simulink model "SIMULINK_ADP_Tracking_R2022b"  (R2023b)
settings: Solver=FixedStepAuto  StartTime=0.0  StopTime=sim_end_time  FixedStep=fixed_step_size  RelTol=1e-3
InitFcn:
  | start_uav_car_10
undefined symbols (not defined in the file): a, act_end, b, battery_threshold, bb, delta_, draw_gif, droneyeeUAV2_NUM, droneyeeUAV3_NUM, droneyeeUAV4_NUM, droneyeeUAV5_NUM, fixed_step_size, k, KD_x, KD_y, kd_z, KDD_x, KDD_y, KI_x, KI_y, ki_z, KII_x, KII_y, KP_x, KP_y, kp_z, KPP_x, KPP_y, lmt, omega, omega_, R, sim_end_time, uav10num, uav1num, uav2num, uav3num, uav4num, uav5num, uav6num, uav7num, uav8num, uav9num, UAV_NUM, Vel_Switch_1, Vel_Switch_10, Vel_Switch_11, Vel_Switch_12, Vel_Switch_13, Vel_Switch_14, Vel_Switch_15, Vel_Switch_16, Vel_Switch_17, Vel_Switch_18, Vel_Switch_19, Vel_Switch_2, Vel_Switch_20, Vel_Switch_3, Vel_Switch_4, Vel_Switch_5 ... (+15)
libraries: simulink x118, aerolibanimutils x1
(part 10 of 11)

== system SIMULINK_ADP_Tracking_R2022b/control system_UAV/Baseline Controller1/Position controller/X-Y ADP tracking controller ==
  Feedback1 : Inport
  Joystick : Inport  Port=2
  p_virtual : Inport  Port=3
  Clock1 : Clock
  Clock2 : Clock
  Clock3 : Clock
  Constant : Constant  Value=5
  Constant1 : Constant  Value=ys_learned
  DMP_ref : MATLAB Function  TreatAsAtomicUnit=on
  Delay : Delay  DelayLength=1  InitialCondition=delta_
  Delay1 : Delay  DelayLength=1  InitialCondition=omega_
  Demux : Demux  Outputs=2
  Demux1 : Demux  Outputs=2
  Derivative : Derivative
  Integrator : Integrator  InitialCondition=W0
  Integrator2 : Integrator  InitialCondition=zeros(2,1)
  Mux1 : Mux  Inputs=3
  Obstacle detection : MATLAB Function  TreatAsAtomicUnit=on
  Saturation : Saturate  UpperLimit=500  LowerLimit=-500
  Saturation1 : Saturate  UpperLimit=100  LowerLimit=-100
  Scope{,1,3..4,6} (5 alike) : Scope
  Scope2 : Scope  NumInputPorts=2
  Scope5 : Scope  NumInputPorts=2
  Terminator : Terminator
  Terminator1 : Terminator
  To Workspace1 : ToWorkspace  VariableName=W  SaveFormat=Timeseries  SampleTime=-1
  To Workspace2 : ToWorkspace  VariableName=Cache1  SampleTime=-1
  XY Graph : Record  FileSettingsInternal="{\"entries\":[{\"content\":{\"excelSettings\":{\"content\":{},\"type\":\"Streamout.ExcelSettings\"}},\"type\":\"Streamout.FileSettingStorage\",\"uuid\":\"\"}],\"packageUris\":[\"http:\\/\\/schema.mathworks.com\\/mf0\\/streamout_blocks\\/R2020a\"],\"version\":\"1.0\"}"  Layout=[1 1]  SignalsInternal="{\"entries\":[{\"content\":{\"signals\":[{\"content\":{\"blockPath\":[],\"dimensions\":[1,1],\"domain\":\"\",\"lineColor\":\"#edb120\",\"port\":1,\"signalID\":1,\"signalName\":\"Demux:1\"},\"type\":\"RecordBlkView.Signal\",\"uuid\":\"\"},{\"content\":{\"blockPath\":[],\"dimensions\":[1,1],\"domain\":\"\",\"lineColor\":\"#7e2f8e\",\"port\":2,\"signalID\":2,\"signalName\":\"Demux:2\"},\"type\":\"RecordBlkView.Signal\",\"uuid\":\"\"}]},\"type\":\"RecordBlkView.InputSignals\",\"uuid\":\"\"}],\"packageUris\":[\"http:\\/\\/schema.mathworks.com\\/mf0\\/streamout_blocks\\/R2020a\"],\"version\":\"1.0\"}"  VisualizationBindings="{\"xyplotplugin\":{\"info\":[{\"series\":[],\"subplotID\":1}]}}"  CompatibilityTag=XY
  adp_tracking : MATLAB Function  TreatAsAtomicUnit=on
  planning output : Scope  NumInputPorts=2
  reference_traj : MATLAB Function  TreatAsAtomicUnit=on
  ux : Outport
  uy : Outport  Port=2
  " p_virtual1" : Outport  Port=3
  wires:
  adp_tracking/1(ux1) -> Scope2/1, ux/1
  Obstacle detection/2(Cache1) -> To Workspace2/1
  Joystick/1 -> adp_tracking/3(Joystick)
  adp_tracking/3(delta_) -> Delay/1
  Delay/1 -> adp_tracking/4(delta_his)
  adp_tracking/4(omega_) -> Scope/1, Delay1/1
  Delay1/1 -> adp_tracking/5(omega_his)
  adp_tracking/5(dW_) -> Saturation/1
  Clock1/1 -> adp_tracking/7(t)
  Integrator/1 -> Scope1/1, To Workspace1/1, adp_tracking/6(W)
  Derivative/1 -> adp_tracking/8(dP_feedback1)
  Saturation/1 -> Integrator/1
  adp_tracking/6(test) -> Scope3/1
  Saturation1/1 -> Derivative/1
  Obstacle detection/1(y) -> Scope4/1, adp_tracking/9(lcoa)
  Demux/1 -> Mux1/1, XY Graph/1, Scope5/1
  Demux/2 -> Mux1/2, XY Graph/2, Scope5/2
  Mux1/1 -> " p_virtual1"/1
  Constant/1 -> Mux1/3
  adp_tracking/2(uy1) -> Scope2/2, uy/1
  reference_traj/1(dp_ref) -> Integrator2/1
  Integrator2/1 -> Terminator/1, reference_traj/2(p_ref)
  Clock2/1 -> reference_traj/1(t)
  reference_traj/2(u_adp) -> Demux1/1
  Demux1/1 -> planning output/1
  Demux1/2 -> planning output/2
  Constant1/1 -> DMP_ref/2(u)
  Clock3/1 -> DMP_ref/1(t)
  Feedback1/1 -> Obstacle detection/1(X), Saturation1/1, adp_tracking/1(P_feedback1)
  p_virtual/1 -> Demux/1, adp_tracking/2(p_virtual1), Scope6/1
  DMP_ref/1(y) -> Terminator1/1

== matlab function SIMULINK_ADP_Tracking_R2022b/control system_car1/Baseline Controller7/MATLAB Function ==
  data: u input; y output; a input
function y = fcn(u,a)
y = satgd(u,a);

== matlab function SIMULINK_ADP_Tracking_R2022b/control system_car1/Baseline Controller8/MATLAB Function ==
  data: u input; y output; a input
function y = fcn(u,a)
y = satgd(u,a);

== matlab function SIMULINK_ADP_Tracking_R2022b/control system_car1/Baseline Controller9/MATLAB Function ==
  data: u input; y output; a input
function y = fcn(u,a)
y = satgd(u,a);

== matlab function SIMULINK_ADP_Tracking_R2022b/防碰撞1/MATLAB Function1 ==
  settings: updateMethod=DISCRETE
  data: u1 input; xd output; u2 input; yd output; zd output; u3 input; u4 input; u5 input; flag input
function [xd,yd,zd] = fcn(u1,u2,u3,u4,u5,flag)

persistent xdd ydd zdd xtt ytt ztt;
k=u4;
totnum =10;
safedist =u3;%安全距离
bang=u5;
xdd=zeros(totnum,1);
ydd=zeros(totnum,1);
zdd=zeros(totnum,1);
xt=zeros(totnum,1);
yt=zeros(totnum,1);
zt=zeros(totnum,1);
vx=xt;
vy=yt;
vz=zt;
xd=xt;
yd=yt;
zd=zt;

for i =1:1:totnum
    xt(i)=u2(12*(i-1)+1);
    yt(i)=u2(12*(i-1)+2);
    zt(i)=u2(12*(i-1)+3);
    vx(i)=u2(12*(i-1)+10);
    vy(i)=u2(12*(i-1)+11);
    vz(i)=u2(12*(i-1)+12);
    xd(i)=u1(4*(i-1)+1);
    yd(i)=u1(4*(i-1)+2);
    zd(i)=u1(4*(i-1)+3);
end
if flag==1
    if isempty(xtt)
        xtt = xt;
        ytt = yt;
        ztt = zt;
    end
    for i =1:1:(totnum-1)
        if (xt(i)==0)&&(yt(i)==0)&&(zt(i)==0)
            continue
        end
        for j=(i+1):1:totnum
            if xt(j)==0 && yt(j)==0 && zt(j)==0
                continue
            end
            dist=(xt(i)-xt(j))^2+(yt(i)-yt(j))^2+(zt(i)-zt(j))^2;
            sqrt_dist=sqrt((xt(i)-xt(j))^2+(yt(i)-yt(j))^2);
            if (dist>0)&&(sqrt(dist)<bang)
                %         xdd(i)=xtt(i);
                %         ydd(i)=ytt(i);
                %         zdd(i)=ztt(i);
                %         xdd(j)=xtt(j);
                %         ydd(j)=ytt(j);
                %         zdd(j)=ztt(j);
                xdd(i)=k*(xt(i)-xt(j))*(safedist-sqrt_dist)/dist;
                ydd(i)=k*(yt(i)-yt(j))*(safedist-sqrt_dist)/dist;
                %         zdd(i)=zt(i)+k*(zt(i)-zt(j))*(safedist-sqrt_dist)/sqrt_dist;
                xdd(j)=-k*(xt(i)-xt(j))*(safedist-sqrt_dist)/dist;
                ydd(j)=-k*(yt(i)-yt(j))*(safedist-sqrt_dist)/dist;
                %         zdd(j)=zt(j)-k*(zt(i)-zt(j))*(safedist-dist)/sqrt_dist;
                
            elseif (sqrt(dist)<safedist)&&(((vx(i)-vx(j))*(xt(i)-xt(j))+...
                    (vy(i)-vy(j))*(yt(i)-yt(j)))<0)
                %         xdd(i)=(xdd(i)+xt(i)+k*(yt(i)-yt(j))*(safedist-sqrt_dist)/dist)/(k*(safedist-sqrt_dist)/dist+1);
                %         ydd(i)=(ydd(i)+yt(i)+k*(xt(j)-xt(i))*(safedist-sqrt_dist)/dist)/(k*(safedist-sqrt_dist)/dist+1);
                %         zdd(i)=zdd(i)+k*(zt(i)-zt(j))*(safedist-sqrt_dist)/sqrt_dist;
                %         xdd(j)=(xdd(j)+xt(j)-k*(yt(i)-yt(j))*(safedist-sqrt_dist)/dist)/(k*(safedist-sqrt_dist)/dist+1);
                %         ydd(j)=(ydd(j)+yt(j)-k*(xt(j)-xt(i))*(safedist-sqrt_dist)/dist)/(k*(safedist-sqrt_dist)/dist+1);
                %         zdd(j)=zdd(j)-k*(zt(i)-zt(j))*(safedist-sqrt_dist)/sqrt_dist;
                %
                %         xdd(i)=(xt(i)+k*(yt(i)-yt(j))*(safedist-sqrt_dist)/dist)/(k*(safedist-sqrt_dist)/dist+1);
                %         ydd(i)=(yt(i)+k*(xt(j)-xt(i))*(safedist-sqrt_dist)/dist)/(k*(safedist-sqrt_dist)/dist+1);
                %         zdd(i)=zdd(i)+k*(zt(i)-zt(j))*(safedist-sqrt_dist)/sqrt_dist;
                %         xdd(j)=(xt(j)-k*(yt(i)-yt(j))*(safedist-sqrt_dist)/dist)/(k*(safedist-sqrt_dist)/dist+1);
                %         ydd(j)=(yt(j)-k*(xt(j)-xt(i))*(safedist-sqrt_dist)/dist)/(k*(safedist-sqrt_dist)/dist+1);
                %         zdd(j)=zdd(j)-k*(zt(i)-zt(j))*(safedist-sqrt_dist)/sqrt_dist;
                
                xdd(i)=(xdd(i)+k*(yt(i)-yt(j))*(safedist-sqrt_dist)/dist);
                ydd(i)=(ydd(i)+k*(xt(j)-xt(i))*(safedist-sqrt_dist)/dist);
                %         zdd(i)=zdd(i)+k*(zt(i)-zt(j))*(safedist-sqrt_dist)/sqrt_dist;
                xdd(j)=(xdd(j)-k*(yt(i)-yt(j))*(safedist-sqrt_dist)/dist);
                ydd(j)=(ydd(j)-k*(xt(j)-xt(i))*(safedist-sqrt_dist)/dist);
                %         zdd(j)=zdd(j)-k*(zt(i)-zt(j))*(safedist-sqrt_dist)/sqrt_dist;
                
            end
        end
        
    end
    
    for m =1:1:totnum
        if (xdd(m) ~= 0)||(ydd(m)~= 0)
            xd(m)=xdd(m)+xt(m);
            yd(m)=ydd(m)+yt(m);
        end
    end
    % zd=zdd;
    
    
end
end

== matlab function SIMULINK_ADP_Tracking_R2022b/CMD_UAV/CMD2/MATLAB Function1 ==
  settings: updateMethod=DISCRETE
  data: x_d input; y_d input; z_d input; timestamp input; x input; y input; z input; battery_status input; sim_time_end input; x_d_ output; battery_threshold input; z_d_for_land input; y_d_ output; z_d_ output; UAV_NUM input
function [x_d_, y_d_, z_d_] = fcn(x_d, y_d, z_d, timestamp, x,y,z,battery_status, sim_time_end,battery_threshold, z_d_for_land, UAV_NUM)
persistent s_x s_y s_z ready_land
if isempty(s_x)
    s_x = x;
end
if isempty(s_y)
    s_y = y;
end
if isempty(s_z)
    s_z = z;
end
if isempty(ready_land)
    ready_land = false;
end
    
battery_low = false;
for i = 1:UAV_NUM
    if battery_status(i) < battery_threshold
        battery_low = true;
        break;
    end
end
if sim_time_end - timestamp < 1
    tello_stop = true;
else
    tello_stop = false;
end
if battery_low || tello_stop
    if ~ready_land
        ready_land = true;
    end
    z_d_ = z_d_for_land;
    x_d_ = s_x;
    y_d_ = s_y;
else
   ready_land = false;
   s_x = x;
   s_y = y;
   x_d_ = x_d;
   y_d_ = y_d;
   z_d_ = z_d;
end

== matlab function SIMULINK_ADP_Tracking_R2022b/control system_car1/Baseline Controller10/MATLAB Function ==
  data: u input; y output; a input
function y = fcn(u,a)
y = satgd(u,a);

== matlab function SIMULINK_ADP_Tracking_R2022b/control system_UAV/Baseline Controller1/Position controller/X-Y ADP tracking controller/Obstacle detection ==
  data: X input; y output; Cache1 output
function [y,Cache1] = LCOA(X)
P_wp1=[10;30];  % target location

% x = X(1:2)-P_wp1;
x = X(1:2);
ro = 2;
ra = ro * 1.5;
rd = ro * 2;
L1 = 0.3; L2 = 0.8; L3 = 0.2;

% zk_ = [10 18; 18 18]-[P_wp1';P_wp1'];
% zk_ = [9-0.5 15; 17-0.5 15];
% zk_ = [9-1 15; 17-1 15];
% zk_ = [9-2 15; 17-2 15];
% zk_ = [1 15; 9 15];
% zk_ = [1.5 15; 8.5 15];
% zk_ = [2 15; 8 15];
% zk_ = [3 12; 7 18];
% zk_ = [3+0.5 15; 9 15];
% zk_ = [9 10; 11.5 25];
% zk_ = [10.5 15; 11.5 25];
zk_ = [11 15; 13 28];

s = 0; ds = [0;0];
beta = 0; dbeta = [0;0];

for i = 1:length(zk_)
    zk = zk_(i,:)';
    dk = norm(x-zk);
    ddk = (x-zk)/dk;
    betak = dk - ro;
    dbetak = ddk;
    
    if dk > rd
        sk = 0;
        dsk = [0;0];
    elseif dk >ra
        sk = L1 + L1 * cos(pi*(dk^2 - ra^2)/(rd^2 - ra^2));
        dsk = -2*pi*dk*ddk*sin(pi*(dk^2 - ra^2)/(rd^2 - ra^2))/(rd^2 - ra^2);
    elseif dk > ro
        sk = L2 + L3 * cos(pi*(dk^2 - ro^2)/(ra^2 - ro^2));
        dsk = -2*pi*dk*ddk*sin(pi*(dk^2 - ro^2)/(ra^2 - ro^2))/(ra^2 - ro^2);
    else
        sk = 1;
        dsk = [0;0];
    end
    ds = ds + dsk; s = s + sk;
    dbeta = dbeta + dbetak;
    beta = beta + betak;
end

mu = 0.1;
Kb = 20000;
% Kb = 20;
% y = Kb * (dsk *(betak + mu) - dbetak * sk)/(betak + mu)^2; 
y = Kb * (ds *(beta + mu) - dbeta * s)/(beta + mu)^2; 


P_wp1=[10;30];  % target location

rrr=[ro;ra;rd];
Cache1=[rrr;P_wp1;zk_(1,:)';zk_(2,:)']; % input for plot111.m

== matlab function SIMULINK_ADP_Tracking_R2022b/control system_UAV/Baseline Controller1/Position controller/X-Y ADP tracking controller/adp_tracking ==
  data: P_feedback1 input; ux1 output; p_virtual1 input; Joystick input; delta_his input; omega_his input; W input; t input; dP_feedback1 input; lcoa input; uy1 output; delta_ output; omega_ output; dW_ output; test output
function [ux1,uy1,delta_,omega_,dW_,test] = adp_tracking(P_feedback1,p_virtual1,Joystick,delta_his,omega_his,W,t,dP_feedback1,lcoa)
% the parameter of 'approaching'

P_wp1=[10;30];  % target location

sampleTime = 1/25;
g = 9.8;
A = zeros(2);
B = eye(2)/g;
Q = 50*eye(2);
R = 100*eye(2);
% R = 500*eye(2);

l = length(W);

dx = dP_feedback1;
% dx = u;

%% ADP Path Planning

% x = P_feedback1 - P_wp1;
x = P_feedback1 - p_virtual1;
x1 = x(1); x2 = x(2);
% phi = [x1^2;x1*x2;x2^2];
% dphi = [2*x1 0; x2 x1; 0 2*x2];
[sig,sig_p] = Staf_Basis(x); % State-following NN basis
dphi = sig_p;
test = norm(dphi);


%% update
umax = 30;
% u_adp = -umax*tanh(0.5/umax*R\B'*dphi'*W);
u_adp = -0.5*R\B'*dphi'*W;
u_safe = -0.5*R\B*lcoa;
u_adp = u_adp + u_safe;% + u_human;
% u_adp = -0.5*R\B'*dphi'*W;
% u_adp = lambda * u_adp + (1-lambda) * u_safe;

if t > 10
%     u = u_adp;
    u = -0.5*R\B'*dphi'*W;
%     u = -umax*tanh(0.5/umax*R\B'*dphi'*W);
else
    u = zeros(2,1);
end
%% ADP nn

omega = dphi*dx;
delta = W'*omega + x'*Q*x + u'*R*u;
rou = 1 + omega'*omega;
delta_ = [delta_his(2:end,:); delta];
omega_ = [omega_his(2:end,:); omega'];

%% Concurrent learning
con_flag = 1;
if con_flag == 1 && t>10
    temp = zeros(l,1);
    for i = 1:length(delta_his)
        omega = omega_(i,:);
        delta = delta_(i,:);
        rou = 1 + omega*omega';
        temp = temp - 1*omega'./rou^2*delta; 
    end
    dW_ = temp;
elseif t>10
        dW_ = - 0.01*omega*delta/rou; 
else
        dW_ = zeros(l,1);
end
%% 输出
% u_adp = u;
ux1 = u_adp(1);
uy1 = u_adp(2);

== matlab function SIMULINK_ADP_Tracking_R2022b/control system_UAV/Baseline Controller1/Position controller/X-Y ADP tracking controller/reference_traj ==
  data: t input; p_ref input; dp_ref output; u_adp output
function [dp_ref,u_adp] = reference_traj(t,p_ref)
g = 9.8;
A = zeros(2);
B = eye(2)/g;
Q = 10*eye(2);
% R = 10*eye(2);
R = 100*eye(2);

P_wp1=[10;30];  % target location
x = p_ref - P_wp1;
x1 = x(1); x2 = x(2);

phi = [x1^2;x1*x2;x2^2];
dphi = [2*x1 0; x2 x1; 0 2*x2];
% [sig,sig_p] = Staf_Basis(x); % State-following NN basis
% dphi = sig_p;
umax = 15;

% W = [69.6962  194.1919  732.3164]';
% W = [240.3627  511.9875  480.4859]';
% W = [626.9039  661.0018  523.60190]';
W = [161.9089  606.9426  710.8552]';
% u_adp = -0.5*R\B'*dphi'*W;
if t > 12
    u_adp = -umax*tanh(0.5/umax*R\B'*dphi'*W);
else
    u_adp = zeros(2,1);
end
dp_ref = A*p_ref + B*u_adp;

== matlab function SIMULINK_ADP_Tracking_R2022b/control system_UAV/Baseline Controller1/Position controller/MATLAB Function ==
  data: x input; p output; y input
function p = fcn(x,y)

p = [x;y];

== matlab function SIMULINK_ADP_Tracking_R2022b/control system_UAV/Baseline Controller1/Position controller/MATLAB Function1 ==
  data: x input; p output; y input
function p = fcn(x,y)

p = [x;y];

== matlab function SIMULINK_ADP_Tracking_R2022b/CMD_UAV/CMD2/Subsystem/MATLAB Function ==
  settings: updateMethod=DISCRETE
  data: timestamp input; uavnum input; x_ output; y_ output; z_ output; switch_flag input; stas input; trj_flag input; form_flag input; avo_flag input
function [x_, y_, z_] = fcn(timestamp, uavnum,switch_flag,stas,trj_flag,form_flag,avo_flag)

[x_,y_,z_]=trjuav(timestamp,uavnum,switch_flag,stas,trj_flag,form_flag,avo_flag);

== matlab function SIMULINK_ADP_Tracking_R2022b/CMD_UAV/CMD1/Subsystem/MATLAB Function ==
  settings: updateMethod=DISCRETE
  data: timestamp input; uavnum input; x_ output; y_ output; z_ output; switch_flag input; stas input; trj_flag input; form_flag input; avo_flag input
function [x_, y_, z_] = fcn(timestamp, uavnum,switch_flag,stas,trj_flag,form_flag,avo_flag)

[x_,y_,z_]=trjuav(timestamp,uavnum,switch_flag,stas,trj_flag,form_flag,avo_flag);

== matlab function SIMULINK_ADP_Tracking_R2022b/CMD_UAV/CMD4/MATLAB Function1 ==
  settings: updateMethod=DISCRETE
  data: x_d input; y_d input; z_d input; timestamp input; x input; y input; z input; battery_status input; sim_time_end input; x_d_ output; battery_threshold input; z_d_for_land input; y_d_ output; z_d_ output; UAV_NUM input
function [x_d_, y_d_, z_d_] = fcn(x_d, y_d, z_d, timestamp, x,y,z,battery_status, sim_time_end,battery_threshold, z_d_for_land, UAV_NUM)
persistent s_x s_y s_z ready_land
if isempty(s_x)
    s_x = x;
end
if isempty(s_y)
    s_y = y;
end
if isempty(s_z)
    s_z = z;
end
if isempty(ready_land)
    ready_land = false;
end
    
battery_low = false;
for i = 1:UAV_NUM
    if battery_status(i) < battery_threshold
        battery_low = true;
        break;
    end
end
if sim_time_end - timestamp < 1
    tello_stop = true;
else
    tello_stop = false;
end
if battery_low || tello_stop
    if ~ready_land
        ready_land = true;
    end
    z_d_ = z_d_for_land;
    x_d_ = s_x;
    y_d_ = s_y;
else
   ready_land = false;
   s_x = x;
   s_y = y;
   x_d_ = x_d;
   y_d_ = y_d;
   z_d_ = z_d;
end

== matlab function SIMULINK_ADP_Tracking_R2022b/CMD_UAV/CMD4/Subsystem/MATLAB Function ==
  settings: updateMethod=DISCRETE
  data: timestamp input; uavnum input; x_ output; y_ output; z_ output; switch_flag input; stas input; trj_flag input; form_flag input; avo_flag input
function [x_, y_, z_] = fcn(timestamp, uavnum,switch_flag,stas,trj_flag,form_flag,avo_flag)

[x_,y_,z_]=trjuav(timestamp,uavnum,switch_flag,stas,trj_flag,form_flag,avo_flag);

== matlab function SIMULINK_ADP_Tracking_R2022b/plot/MATLAB Function ==
  data: x1 input; y1 input; z1 input; x2 input; y2 input; z2 input; x3 input; y3 input; z3 input; x4 input; y4 input; z4 input; x5 input; y5 input; z5 input; x6 input; y6 input; z6 input; x7 input; y7 input; z7 input; x8 input; y8 input; z8 input; x9 input; y9 input; z9 input; x10 input; y10 input; z10 input; x11 input; y11 input; z11 input; x12 input; y12 input; z12 input; x13 input; y13 input; z13 input; x14 input; y14 input; z14 input; x15 input; y15 input; z15 input; x16 input; y16 input; z16 input; x17 input; y17 input; z17 input; x18 input; y18 input; z18 input; x19 input; y19 input; z19 input; x20 input; y20 input; z20 input; x21 input; y21 input; z21 input; x22 input; y22 input; z22 input; x23 input; y23 input; z23 input; x24 input; y24 input; z24 input; time_step input; act_end input; XMIN input; XMAX input; YMIN input; YMAX input; ZMIN input; ZMAX input; a input; b input; k input; bb input; w1 input; w2 input; draw_gif input
function f_eight_shaped(x1, y1, z1, x2, y2, z2, x3, y3, z3,x4, y4, z4, x5, y5, z5, x6, y6, z6, x7, y7, z7,x8, y8, z8,x9, y9, z9,x10,y10,z10,x11, y11, z11, x12, y12, z12, x13, y13, z13,x14, y14, z14, x15, y15, z15, x16, y16, z16, x17, y17, z17,x18, y18, z18,x19, y19, z19,x20,y20,z20,x21, y21, z21, x22, y22, z22, x23, y23, z23,x24, y24, z24,time_step, act_end, XMIN,XMAX, YMIN, YMAX, ZMIN, ZMAX, a, b, k, bb, w1, w2,draw_gif)

% persistent index
% if isempty(index)
%     index = 0;
% end
% length = 8000;
% persistent posd_x  posd_y posd_z
% if isempty(posd_x)
%     posd_x = zeros(length,1);
% end
% if isempty(posd_y)
%     posd_y = zeros(length,1);
% end
% if isempty(posd_z)
%     posd_z = zeros(length,1);
% end
% 
% index = index + 1;
% if index <= 1
%     axis([XMIN*1.2 XMAX*1.2 YMIN*1.2 YMAX*1.2 ZMIN*0.5 ZMAX*1.2]);
%     xlabel('X(m)');
%     ylabel('Y(m)');
%     zlabel('Z(m)');
%     box on;
%     i= 0;
%     for t = 0:time_step:act_end
%         i = i+1;
%         posd_x(i) = a*cos(w1*t);
%         posd_y(i) = b*sin(w2*t);
%         posd_z(i) = k*posd_x(i) + bb;
%     end
% else
    cla;
    hold on
    %data_num = floor(act_end/time_step);
%     plot3(posd_x(1:data_num), posd_y(1:data_num), posd_z(1:data_num));
    plot3(x1,y1,z1,'ro');
    plot3(x2,y2,z2,'g*');
    plot3(x3,y3,z3,'bo');
    plot3(x4,y4,z4,'y*');
    plot3(x5,y5,z5,'co');
    plot3(x6,y6,z6,'m*');
    plot3(x7,y7,z7,'ko');
    plot3(x8,y8,z8,'r*');
    plot3(x9,y9,z9,'cp');
    plot3(x10,y10,z10,'bs');
%     coder.extrinsic('getframe')
%     if draw_gif
%          frame=getframe(gcf);
%          imind=frame2im(frame);
%          [imind,cm] = rgb2ind(imind,256);
%          if index <=2
%              imwrite(imind,cm,'eight-shaped.gif','gif', 'Loopcount',inf,'DelayTime',time_step);
%          else
%              imwrite(imind,cm,'eight-shaped.gif','gif','WriteMode','append','DelayTime',time_step);
%          end
%     end
end

== matlab function SIMULINK_ADP_Tracking_R2022b/CMD_UAV/CMD5/MATLAB Function1 ==
  settings: updateMethod=DISCRETE
  data: x_d input; y_d input; z_d input; timestamp input; x input; y input; z input; battery_status input; sim_time_end input; x_d_ output; battery_threshold input; z_d_for_land input; y_d_ output; z_d_ output; UAV_NUM input
function [x_d_, y_d_, z_d_] = fcn(x_d, y_d, z_d, timestamp, x,y,z,battery_status, sim_time_end,battery_threshold, z_d_for_land, UAV_NUM)
persistent s_x s_y s_z ready_land
if isempty(s_x)
    s_x = x;
end
if isempty(s_y)
    s_y = y;
end
if isempty(s_z)
    s_z = z;
end
if isempty(ready_land)
    ready_land = false;
end
    
battery_low = false;
for i = 1:UAV_NUM
    if battery_status(i) < battery_threshold
        battery_low = true;
        break;
    end
end
if sim_time_end - timestamp < 1
    tello_stop = true;
else
    tello_stop = false;
end
if battery_low || tello_stop
    if ~ready_land
        ready_land = true;
    end
    z_d_ = z_d_for_land;
    x_d_ = s_x;
    y_d_ = s_y;
else
   ready_land = false;
   s_x = x;
   s_y = y;
   x_d_ = x_d;
   y_d_ = y_d;
   z_d_ = z_d;
end

== matlab function SIMULINK_ADP_Tracking_R2022b/CMD_UAV/CMD5/Subsystem/MATLAB Function ==
  settings: updateMethod=DISCRETE
  data: timestamp input; uavnum input; x_ output; y_ output; z_ output; switch_flag input; stas input; trj_flag input; form_flag input; avo_flag input
function [x_, y_, z_] = fcn(timestamp, uavnum,switch_flag,stas,trj_flag,form_flag,avo_flag)

[x_,y_,z_]=trjuav(timestamp,uavnum,switch_flag,stas,trj_flag,form_flag,avo_flag);

== matlab function SIMULINK_ADP_Tracking_R2022b/CMD_UAV/CMD3/Subsystem/MATLAB Function ==
  settings: updateMethod=DISCRETE
  data: timestamp input; uavnum input; x_ output; y_ output; z_ output; switch_flag input; stas input; trj_flag input; form_flag input; avo_flag input
function [x_, y_, z_] = fcn(timestamp, uavnum,switch_flag,stas,trj_flag,form_flag,avo_flag)

[x_,y_,z_]=trjuav(timestamp,uavnum,switch_flag,stas,trj_flag,form_flag,avo_flag);

== matlab function SIMULINK_ADP_Tracking_R2022b/CMD_car1/CMD1/MATLAB Function1 ==
  settings: updateMethod=DISCRETE
  data: x_d input; y_d input; z_d input; timestamp input; x input; y input; z input; battery_status input; sim_time_end input; x_d_ output; battery_threshold input; z_d_for_land input; y_d_ output; z_d_ output; UAV_NUM input
function [x_d_, y_d_, z_d_] = fcn(x_d, y_d, z_d, timestamp, x,y,z,battery_status, sim_time_end,battery_threshold, z_d_for_land, UAV_NUM)
persistent s_x s_y s_z ready_land
if isempty(s_x)
    s_x = x;
end
if isempty(s_y)
    s_y = y;
end
if isempty(s_z)
    s_z = z;
end
if isempty(ready_land)
    ready_land = false;
end
    
battery_low = false;
for i = 1:UAV_NUM
    if battery_status(i) < battery_threshold
        battery_low = true;
        break;
    end
end
if sim_time_end - timestamp < 1
    tello_stop = true;
else
    tello_stop = false;
end
if battery_low || tello_stop
    if ~ready_land
        ready_land = true;
    end
    z_d_ = z_d_for_land;
    x_d_ = s_x;
    y_d_ = s_y;
else
   ready_land = false;
   s_x = x;
   s_y = y;
   x_d_ = x_d;
   y_d_ = y_d;
   z_d_ = z_d;
end

== matlab function SIMULINK_ADP_Tracking_R2022b/control system_UAV/Baseline Controller1/MATLAB Function ==
  data: u input; y output; a input
function y = fcn(u,a)
y = satgd(u,a);

== matlab function SIMULINK_ADP_Tracking_R2022b/CMD_UAV/CMD3/MATLAB Function1 ==
  settings: updateMethod=DISCRETE
  data: x_d input; y_d input; z_d input; timestamp input; x input; y input; z input; battery_status input; sim_time_end input; x_d_ output; battery_threshold input; z_d_for_land input; y_d_ output; z_d_ output; UAV_NUM input
function [x_d_, y_d_, z_d_] = fcn(x_d, y_d, z_d, timestamp, x,y,z,battery_status, sim_time_end,battery_threshold, z_d_for_land, UAV_NUM)
persistent s_x s_y s_z ready_land
if isempty(s_x)
    s_x = x;
end
if isempty(s_y)
    s_y = y;
end
if isempty(s_z)
    s_z = z;
end
if isempty(ready_land)
    ready_land = false;
end
    
battery_low = false;
for i = 1:UAV_NUM
    if battery_status(i) < battery_threshold
        battery_low = true;
        break;
    end
end
if sim_time_end - timestamp < 1
    tello_stop = true;
else
    tello_stop = false;
end
if battery_low || tello_stop
    if ~ready_land
        ready_land = true;
    end
    z_d_ = z_d_for_land;
    x_d_ = s_x;
    y_d_ = s_y;
else
   ready_land = false;
   s_x = x;
   s_y = y;
   x_d_ = x_d;
   y_d_ = y_d;
   z_d_ = z_d;
end

== matlab function SIMULINK_ADP_Tracking_R2022b/CMD_car1/CMD1/Subsystem/MATLAB Function ==
  settings: updateMethod=DISCRETE
  data: timestamp input; uavnum input; x_ output; y_ output; z_ output; switch_flag input; stas input; trj_flag input; form_flag input; avo_flag input
function [x_, y_, z_] = fcn(timestamp, uavnum,switch_flag,stas,trj_flag,form_flag,avo_flag)

[x_,y_,z_]=trjcar(timestamp,uavnum,switch_flag,stas,trj_flag,form_flag,avo_flag);

== matlab function SIMULINK_ADP_Tracking_R2022b/control system_UAV/Baseline Controller1/Position controller/X-Y ADP tracking controller/DMP_ref ==
  data: t input; u input; y output
function y = fcn(t,u)
N = length(u);
if t < 12
    y = [0,0]';
elseif t < 12+N*0.01 -1
    i = floor((t-12)/0.01)+1;
    y = (u(i,:)-u(1,:))';
else
    y = (u(end,:)-u(1,:))';
end
% y = y';

== matlab function SIMULINK_ADP_Tracking_R2022b/CMD_car1/CMD10/MATLAB Function1 ==
  settings: updateMethod=DISCRETE
  data: x_d input; y_d input; z_d input; timestamp input; x input; y input; z input; battery_status input; sim_time_end input; x_d_ output; battery_threshold input; z_d_for_land input; y_d_ output; z_d_ output; UAV_NUM input
function [x_d_, y_d_, z_d_] = fcn(x_d, y_d, z_d, timestamp, x,y,z,battery_status, sim_time_end,battery_threshold, z_d_for_land, UAV_NUM)
persistent s_x s_y s_z ready_land
if isempty(s_x)
    s_x = x;
end
if isempty(s_y)
    s_y = y;
end
if isempty(s_z)
    s_z = z;
end
if isempty(ready_land)
    ready_land = false;
end
    
battery_low = false;
for i = 1:UAV_NUM
    if battery_status(i) < battery_threshold
        battery_low = true;
        break;
    end
end
if sim_time_end - timestamp < 1
    tello_stop = true;
else
    tello_stop = false;
end
if battery_low || tello_stop
    if ~ready_land
        ready_land = true;
    end
    z_d_ = z_d_for_land;
    x_d_ = s_x;
    y_d_ = s_y;
else
   ready_land = false;
   s_x = x;
   s_y = y;
   x_d_ = x_d;
   y_d_ = y_d;
   z_d_ = z_d;
end

== matlab function SIMULINK_ADP_Tracking_R2022b/CMD_UAV/CMD1/MATLAB Function1 ==
  settings: updateMethod=DISCRETE
  data: x_d input; y_d input; z_d input; timestamp input; x input; y input; z input; battery_status input; sim_time_end input; x_d_ output; battery_threshold input; z_d_for_land input; y_d_ output; z_d_ output; UAV_NUM input
function [x_d_, y_d_, z_d_] = fcn(x_d, y_d, z_d, timestamp, x,y,z,battery_status, sim_time_end,battery_threshold, z_d_for_land, UAV_NUM)
persistent s_x s_y s_z ready_land
if isempty(s_x)
    s_x = x;
end
if isempty(s_y)
    s_y = y;
end
if isempty(s_z)
    s_z = z;
end
if isempty(ready_land)
    ready_land = false;
end
    
battery_low = false;
for i = 1:UAV_NUM
    if battery_status(i) < battery_threshold
        battery_low = true;
        break;
    end
end
if sim_time_end - timestamp < 1
    tello_stop = true;
else
    tello_stop = false;
end
if battery_low || tello_stop
    if ~ready_land
        ready_land = true;
    end
    z_d_ = z_d_for_land;
    x_d_ = s_x;
    y_d_ = s_y;
else
   ready_land = false;
   s_x = x;
   s_y = y;
   x_d_ = x_d;
   y_d_ = y_d;
   z_d_ = z_d;
end

== matlab function SIMULINK_ADP_Tracking_R2022b/CMD_car1/CMD10/Subsystem/MATLAB Function ==
  settings: updateMethod=DISCRETE
  data: timestamp input; uavnum input; x_ output; y_ output; z_ output; switch_flag input; stas input; trj_flag input; form_flag input; avo_flag input
function [x_, y_, z_] = fcn(timestamp, uavnum,switch_flag,stas,trj_flag,form_flag,avo_flag)

[x_,y_,z_]=trjcar(timestamp,uavnum,switch_flag,stas,trj_flag,form_flag,avo_flag);

== matlab function SIMULINK_ADP_Tracking_R2022b/CMD_car1/CMD2/MATLAB Function1 ==
  settings: updateMethod=DISCRETE
  data: x_d input; y_d input; z_d input; timestamp input; x input; y input; z input; battery_status input; sim_time_end input; x_d_ output; battery_threshold input; z_d_for_land input; y_d_ output; z_d_ output; UAV_NUM input
function [x_d_, y_d_, z_d_] = fcn(x_d, y_d, z_d, timestamp, x,y,z,battery_status, sim_time_end,battery_threshold, z_d_for_land, UAV_NUM)
persistent s_x s_y s_z ready_land
if isempty(s_x)
    s_x = x;
end
if isempty(s_y)
    s_y = y;
end
if isempty(s_z)
    s_z = z;
end
if isempty(ready_land)
    ready_land = false;
end
    
battery_low = false;
for i = 1:UAV_NUM
    if battery_status(i) < battery_threshold
        battery_low = true;
        break;
    end
end
if sim_time_end - timestamp < 1
    tello_stop = true;
else
    tello_stop = false;
end
if battery_low || tello_stop
    if ~ready_land
        ready_land = true;
    end
    z_d_ = z_d_for_land;
    x_d_ = s_x;
    y_d_ = s_y;
else
   ready_land = false;
   s_x = x;
   s_y = y;
   x_d_ = x_d;
   y_d_ = y_d;
   z_d_ = z_d;
end

== matlab function SIMULINK_ADP_Tracking_R2022b/CMD_car1/CMD2/Subsystem/MATLAB Function ==
  settings: updateMethod=DISCRETE
  data: timestamp input; uavnum input; x_ output; y_ output; z_ output; switch_flag input; stas input; trj_flag input; form_flag input; avo_flag input
function [x_, y_, z_] = fcn(timestamp, uavnum,switch_flag,stas,trj_flag,form_flag,avo_flag)

[x_,y_,z_]=trjcar(timestamp,uavnum,switch_flag,stas,trj_flag,form_flag,avo_flag);

== matlab function SIMULINK_ADP_Tracking_R2022b/CMD_car1/CMD3/MATLAB Function1 ==
  settings: updateMethod=DISCRETE
  data: x_d input; y_d input; z_d input; timestamp input; x input; y input; z input; battery_status input; sim_time_end input; x_d_ output; battery_threshold input; z_d_for_land input; y_d_ output; z_d_ output; UAV_NUM input
function [x_d_, y_d_, z_d_] = fcn(x_d, y_d, z_d, timestamp, x,y,z,battery_status, sim_time_end,battery_threshold, z_d_for_land, UAV_NUM)
persistent s_x s_y s_z ready_land
if isempty(s_x)
    s_x = x;
end
if isempty(s_y)
    s_y = y;
end
if isempty(s_z)
    s_z = z;
end
if isempty(ready_land)
    ready_land = false;
end
    
battery_low = false;
for i = 1:UAV_NUM
    if battery_status(i) < battery_threshold
        battery_low = true;
        break;
    end
end
if sim_time_end - timestamp < 1
    tello_stop = true;
else
    tello_stop = false;
end
if battery_low || tello_stop
    if ~ready_land
        ready_land = true;
    end
    z_d_ = z_d_for_land;
    x_d_ = s_x;
    y_d_ = s_y;
else
   ready_land = false;
   s_x = x;
   s_y = y;
   x_d_ = x_d;
   y_d_ = y_d;
   z_d_ = z_d;
end

== matlab function SIMULINK_ADP_Tracking_R2022b/CMD_car1/CMD3/Subsystem/MATLAB Function ==
  settings: updateMethod=DISCRETE
  data: timestamp input; uavnum input; x_ output; y_ output; z_ output; switch_flag input; stas input; trj_flag input; form_flag input; avo_flag input
function [x_, y_, z_] = fcn(timestamp, uavnum,switch_flag,stas,trj_flag,form_flag,avo_flag)

[x_,y_,z_]=trjcar(timestamp,uavnum,switch_flag,stas,trj_flag,form_flag,avo_flag);

== matlab function SIMULINK_ADP_Tracking_R2022b/CMD_UAV/CMD6/MATLAB Function1 ==
  settings: updateMethod=DISCRETE
  data: x_d input; y_d input; z_d input; timestamp input; x input; y input; z input; battery_status input; sim_time_end input; x_d_ output; battery_threshold input; z_d_for_land input; y_d_ output; z_d_ output; UAV_NUM input
function [x_d_, y_d_, z_d_] = fcn(x_d, y_d, z_d, timestamp, x,y,z,battery_status, sim_time_end,battery_threshold, z_d_for_land, UAV_NUM)
persistent s_x s_y s_z ready_land
if isempty(s_x)
    s_x = x;
end
if isempty(s_y)
    s_y = y;
end
if isempty(s_z)
    s_z = z;
end
if isempty(ready_land)
    ready_land = false;
end
    
battery_low = false;
for i = 1:UAV_NUM
    if battery_status(i) < battery_threshold
        battery_low = true;
        break;
    end
end
if sim_time_end - timestamp < 1
    tello_stop = true;
else
    tello_stop = false;
end
if battery_low || tello_stop
    if ~ready_land
        ready_land = true;
    end
    z_d_ = z_d_for_land;
    x_d_ = s_x;
    y_d_ = s_y;
else
   ready_land = false;
   s_x = x;
   s_y = y;
   x_d_ = x_d;
   y_d_ = y_d;
   z_d_ = z_d;
end

== matlab function SIMULINK_ADP_Tracking_R2022b/CMD_car1/CMD4/MATLAB Function1 ==
  settings: updateMethod=DISCRETE
  data: x_d input; y_d input; z_d input; timestamp input; x input; y input; z input; battery_status input; sim_time_end input; x_d_ output; battery_threshold input; z_d_for_land input; y_d_ output; z_d_ output; UAV_NUM input
function [x_d_, y_d_, z_d_] = fcn(x_d, y_d, z_d, timestamp, x,y,z,battery_status, sim_time_end,battery_threshold, z_d_for_land, UAV_NUM)
persistent s_x s_y s_z ready_land
if isempty(s_x)
    s_x = x;
end
if isempty(s_y)
    s_y = y;
end
if isempty(s_z)
    s_z = z;
end
if isempty(ready_land)
    ready_land = false;
end
    
battery_low = false;
for i = 1:UAV_NUM
    if battery_status(i) < battery_threshold
        battery_low = true;
        break;
    end
end
if sim_time_end - timestamp < 1
    tello_stop = true;
else
    tello_stop = false;
end
if battery_low || tello_stop
    if ~ready_land
        ready_land = true;
    end
    z_d_ = z_d_for_land;
    x_d_ = s_x;
    y_d_ = s_y;
else
   ready_land = false;
   s_x = x;
   s_y = y;
   x_d_ = x_d;
   y_d_ = y_d;
   z_d_ = z_d;
end

== matlab function SIMULINK_ADP_Tracking_R2022b/CMD_car1/CMD4/Subsystem/MATLAB Function ==
  settings: updateMethod=DISCRETE
  data: timestamp input; uavnum input; x_ output; y_ output; z_ output; switch_flag input; stas input; trj_flag input; form_flag input; avo_flag input
function [x_, y_, z_] = fcn(timestamp, uavnum,switch_flag,stas,trj_flag,form_flag,avo_flag)

[x_,y_,z_]=trjcar(timestamp,uavnum,switch_flag,stas,trj_flag,form_flag,avo_flag);

== matlab function SIMULINK_ADP_Tracking_R2022b/CMD_car1/CMD5/MATLAB Function1 ==
  settings: updateMethod=DISCRETE
  data: x_d input; y_d input; z_d input; timestamp input; x input; y input; z input; battery_status input; sim_time_end input; x_d_ output; battery_threshold input; z_d_for_land input; y_d_ output; z_d_ output; UAV_NUM input
function [x_d_, y_d_, z_d_] = fcn(x_d, y_d, z_d, timestamp, x,y,z,battery_status, sim_time_end,battery_threshold, z_d_for_land, UAV_NUM)
persistent s_x s_y s_z ready_land
if isempty(s_x)
    s_x = x;
end
if isempty(s_y)
    s_y = y;
end
if isempty(s_z)
    s_z = z;
end
if isempty(ready_land)
    ready_land = false;
end
    
battery_low = false;
for i = 1:UAV_NUM
    if battery_status(i) < battery_threshold
        battery_low = true;
        break;
    end
end
if sim_time_end - timestamp < 1
    tello_stop = true;
else
    tello_stop = false;
end
if battery_low || tello_stop
    if ~ready_land
        ready_land = true;
    end
    z_d_ = z_d_for_land;
    x_d_ = s_x;
    y_d_ = s_y;
else
   ready_land = false;
   s_x = x;
   s_y = y;
   x_d_ = x_d;
   y_d_ = y_d;
   z_d_ = z_d;
end

== matlab function SIMULINK_ADP_Tracking_R2022b/CMD_car1/CMD5/Subsystem/MATLAB Function ==
  settings: updateMethod=DISCRETE
  data: timestamp input; uavnum input; x_ output; y_ output; z_ output; switch_flag input; stas input; trj_flag input; form_flag input; avo_flag input
function [x_, y_, z_] = fcn(timestamp, uavnum,switch_flag,stas,trj_flag,form_flag,avo_flag)

[x_,y_,z_]=trjcar(timestamp,uavnum,switch_flag,stas,trj_flag,form_flag,avo_flag);

== matlab function SIMULINK_ADP_Tracking_R2022b/CMD_car1/CMD6/MATLAB Function1 ==
  settings: updateMethod=DISCRETE
  data: x_d input; y_d input; z_d input; timestamp input; x input; y input; z input; battery_status input; sim_time_end input; x_d_ output; battery_threshold input; z_d_for_land input; y_d_ output; z_d_ output; UAV_NUM input
function [x_d_, y_d_, z_d_] = fcn(x_d, y_d, z_d, timestamp, x,y,z,battery_status, sim_time_end,battery_threshold, z_d_for_land, UAV_NUM)
persistent s_x s_y s_z ready_land
if isempty(s_x)
    s_x = x;
end
if isempty(s_y)
    s_y = y;
end
if isempty(s_z)
    s_z = z;
end
if isempty(ready_land)
    ready_land = false;
end
    
battery_low = false;
for i = 1:UAV_NUM
    if battery_status(i) < battery_threshold
        battery_low = true;
        break;
    end
end
if sim_time_end - timestamp < 1
    tello_stop = true;
else
    tello_stop = false;
end
if battery_low || tello_stop
    if ~ready_land
        ready_land = true;
    end
    z_d_ = z_d_for_land;
    x_d_ = s_x;
    y_d_ = s_y;
else
   ready_land = false;
   s_x = x;
   s_y = y;
   x_d_ = x_d;
   y_d_ = y_d;
   z_d_ = z_d;
end

== matlab function SIMULINK_ADP_Tracking_R2022b/control system_UAV/MATLAB Function ==
  data: u input; y output
function y = fcn(u)
plot(u(1),u(2),"*");
hold on;
y = u;

== matlab function SIMULINK_ADP_Tracking_R2022b/防碰撞2/MATLAB Function ==
  settings: updateMethod=DISCRETE
  data: u1 input; xd output; u2 input; yd output; zd output; u3 input; u4 input; u5 input; flag input
function [xd,yd,zd] = fcn(u1,u2,u3,u4,u5,flag)
persistent xdd ydd zdd xtt ytt ztt;
k=u4;
totnum =10;
safedist =u3;%安全距离的平方
bang=u5;
xdd=zeros(totnum,1);
ydd=zeros(totnum,1);
zdd=zeros(totnum,1);
xt=zeros(totnum,1);
yt=zeros(totnum,1);
zt=zeros(totnum,1);
vx=xt;
vy=yt;
vz=zt;
xd=xt;
yd=yt;
zd=zt;
for i =1:1:totnum
    xt(i)=u2(12*(i-1)+1);
    yt(i)=u2(12*(i-1)+2);
    zt(i)=u2(12*(i-1)+3);
    xd(i)=u1(6*(i-1)+1);
    yd(i)=u1(6*(i-1)+2);
    zd(i)=u1(6*(i-1)+3);
    vx(i)=u2(12*(i-1)+10);
    vy(i)=u2(12*(i-1)+11);
    vz(i)=u2(12*(i-1)+12);
end
if flag==1
if isempty(xt)
    xtt = xt;
    ytt = yt;
    ztt = zt;
end
for i =1:1:(totnum-1)
    if xt(i)==0&&yt(i)==0&&zt(i)==0
        break
    end
    for j=(i+1):1:totnum
        if xt(j)==0&&yt(j)==0&&zt(j)==0
        break
        end
        dist=((xt(i)-xt(j))^2+(yt(i)-yt(j))^2+(zt(i)-zt(j))^2);
        sqrt_dist=sqrt((xt(i)-xt(j))^2+(yt(i)-yt(j))^2);
    if (dist>0)&&(sqrt(dist)<=bang)
%         xd(i)=xt(i);
%         yd(i)=yt(i);
%         zd(i)=0; %zt(i);
%         xd(j)=xt(j);
%         yd(j)=yt(j);
%         zd(j)=zt(j);        
%         xd(i)=xd(i)+k*(xt(i)-xt(j))*(safedist-dist);
%         yd(i)=yd(i)+k*(yt(i)-yt(j))*(safedist-dist);
        xdd(i)=xdd(i)+k*(xt(i)-xt(j))*(safedist-dist);
        ydd(i)=ydd(i)+k*(yt(i)-yt(j))*(safedist-dist);
%         zd(i)=zd(i)+k*(zt(i)-zt(j))*(safedist-dist);
%         xd(j)=xd(j)-k*(xt(i)-xt(j))*(safedist-dist);
%         yd(j)=yd(j)-k*(yt(i)-yt(j))*(safedist-dist);
        xdd(j)=xdd(j)-k*(xt(i)-xt(j))*(safedist-dist);
        ydd(j)=ydd(j)-k*(yt(i)-yt(j))*(safedist-dist);
%         zd(j)=zd(j)-k*(zt(i)-zt(j))*(safedist-dist);
     elseif (sqrt(dist)<safedist)&&(((vx(i)-vx(j))*(xt(i)-xt(j))+...
             (vy(i)-vy(j))*(yt(i)-yt(j)))<0)
%         dist=dist-bang;
%         xd(i)=xd(i)+k*(yt(i)-yt(j))*(safedist-dist);
%         yd(i)=yd(i)+k*(xt(j)-xt(i))*(safedist-dist);
        xdd(i)=xdd(i)+k*(yt(i)-yt(j))*(safedist-sqrt_dist)/sqrt_dist/sqrt_dist;
        ydd(i)=ydd(i)+k*(xt(j)-xt(i))*(safedist-sqrt_dist)/sqrt_dist/sqrt_dist;
%         zd(i)=zd(i)+k*(zt(i)-zt(j))*(safedist-dist);
%         xd(j)=xd(j)-k*(yt(i)-yt(j))*(safedist-dist);
%         yd(j)=yd(j)-k*(xt(j)-xt(i))*(safedist-dist);
        xdd(j)=xdd(j)-k*(yt(i)-yt(j))*(safedist-sqrt_dist)/sqrt_dist/sqrt_dist;
        ydd(j)=ydd(j)-k*(xt(j)-xt(i))*(safedist-sqrt_dist)/sqrt_dist/sqrt_dist;
%         zd(j)=zd(j)-k*(zt(i)-zt(j))*(safedist-dist);
        
    end
    end
end
xd=xd+xdd;
yd=yd+ydd;
% zd=zdd;
end

== matlab function SIMULINK_ADP_Tracking_R2022b/control system_UAV/Baseline Controller3/MATLAB Function ==
  data: u input; y output; a input
function y = fcn(u,a)
y = satgd(u,a);

== matlab function SIMULINK_ADP_Tracking_R2022b/CMD_car1/CMD6/Subsystem/MATLAB Function ==
  settings: updateMethod=DISCRETE
  data: timestamp input; uavnum input; x_ output; y_ output; z_ output; switch_flag input; stas input; trj_flag input; form_flag input; avo_flag input
function [x_, y_, z_] = fcn(timestamp, uavnum,switch_flag,stas,trj_flag,form_flag,avo_flag)

[x_,y_,z_]=trjcar(timestamp,uavnum,switch_flag,stas,trj_flag,form_flag,avo_flag);

== matlab function SIMULINK_ADP_Tracking_R2022b/control system_UAV/Baseline Controller4/MATLAB Function ==
  data: u input; y output; a input
function y = fcn(u,a)
y = satgd(u,a);

== matlab function SIMULINK_ADP_Tracking_R2022b/CMD_car1/CMD7/MATLAB Function1 ==
  settings: updateMethod=DISCRETE
  data: x_d input; y_d input; z_d input; timestamp input; x input; y input; z input; battery_status input; sim_time_end input; x_d_ output; battery_threshold input; z_d_for_land input; y_d_ output; z_d_ output; UAV_NUM input
function [x_d_, y_d_, z_d_] = fcn(x_d, y_d, z_d, timestamp, x,y,z,battery_status, sim_time_end,battery_threshold, z_d_for_land, UAV_NUM)
persistent s_x s_y s_z ready_land
if isempty(s_x)
    s_x = x;
end
if isempty(s_y)
    s_y = y;
end
if isempty(s_z)
    s_z = z;
end
if isempty(ready_land)
    ready_land = false;
end
    
battery_low = false;
for i = 1:UAV_NUM
    if battery_status(i) < battery_threshold
        battery_low = true;
        break;
    end
end
if sim_time_end - timestamp < 1
    tello_stop = true;
else
    tello_stop = false;
end
if battery_low || tello_stop
    if ~ready_land
        ready_land = true;
    end
    z_d_ = z_d_for_land;
    x_d_ = s_x;
    y_d_ = s_y;
else
   ready_land = false;
   s_x = x;
   s_y = y;
   x_d_ = x_d;
   y_d_ = y_d;
   z_d_ = z_d;
end

== matlab function SIMULINK_ADP_Tracking_R2022b/CMD_UAV/CMD6/Subsystem/MATLAB Function ==
  settings: updateMethod=DISCRETE
  data: timestamp input; uavnum input; x_ output; y_ output; z_ output; switch_flag input; stas input; trj_flag input; form_flag input; avo_flag input
function [x_, y_, z_] = fcn(timestamp, uavnum,switch_flag,stas,trj_flag,form_flag,avo_flag)

[x_,y_,z_]=trjuav(timestamp,uavnum,switch_flag,stas,trj_flag,form_flag,avo_flag);

== matlab function SIMULINK_ADP_Tracking_R2022b/CMD_UAV/CMD7/MATLAB Function1 ==
  settings: updateMethod=DISCRETE
  data: x_d input; y_d input; z_d input; timestamp input; x input; y input; z input; battery_status input; sim_time_end input; x_d_ output; battery_threshold input; z_d_for_land input; y_d_ output; z_d_ output; UAV_NUM input
function [x_d_, y_d_, z_d_] = fcn(x_d, y_d, z_d, timestamp, x,y,z,battery_status, sim_time_end,battery_threshold, z_d_for_land, UAV_NUM)
persistent s_x s_y s_z ready_land
if isempty(s_x)
    s_x = x;
end
if isempty(s_y)
    s_y = y;
end
if isempty(s_z)
    s_z = z;
end
if isempty(ready_land)
    ready_land = false;
end
    
battery_low = false;
for i = 1:UAV_NUM
    if battery_status(i) < battery_threshold
        battery_low = true;
        break;
    end
end
if sim_time_end - timestamp < 1
    tello_stop = true;
else
    tello_stop = false;
end
if battery_low || tello_stop
    if ~ready_land
        ready_land = true;
    end
    z_d_ = z_d_for_land;
    x_d_ = s_x;
    y_d_ = s_y;
else
   ready_land = false;
   s_x = x;
   s_y = y;
   x_d_ = x_d;
   y_d_ = y_d;
   z_d_ = z_d;
end

== matlab function SIMULINK_ADP_Tracking_R2022b/CMD_UAV/CMD7/Subsystem/MATLAB Function ==
  settings: updateMethod=DISCRETE
  data: timestamp input; uavnum input; x_ output; y_ output; z_ output; switch_flag input; stas input; trj_flag input; form_flag input; avo_flag input
function [x_, y_, z_] = fcn(timestamp, uavnum,switch_flag,stas,trj_flag,form_flag,avo_flag)

[x_,y_,z_]=trjuav(timestamp,uavnum,switch_flag,stas,trj_flag,form_flag,avo_flag);

== matlab function SIMULINK_ADP_Tracking_R2022b/CMD_UAV/CMD8/MATLAB Function1 ==
  settings: updateMethod=DISCRETE
  data: x_d input; y_d input; z_d input; timestamp input; x input; y input; z input; battery_status input; sim_time_end input; x_d_ output; battery_threshold input; z_d_for_land input; y_d_ output; z_d_ output; UAV_NUM input
function [x_d_, y_d_, z_d_] = fcn(x_d, y_d, z_d, timestamp, x,y,z,battery_status, sim_time_end,battery_threshold, z_d_for_land, UAV_NUM)
persistent s_x s_y s_z ready_land
if isempty(s_x)
    s_x = x;
end
if isempty(s_y)
    s_y = y;
end
if isempty(s_z)
    s_z = z;
end
if isempty(ready_land)
    ready_land = false;
end
    
battery_low = false;
for i = 1:UAV_NUM
    if battery_status(i) < battery_threshold
        battery_low = true;
        break;
    end
end
if sim_time_end - timestamp < 1
    tello_stop = true;
else
    tello_stop = false;
end
if battery_low || tello_stop
    if ~ready_land
        ready_land = true;
    end
    z_d_ = z_d_for_land;
    x_d_ = s_x;
    y_d_ = s_y;
else
   ready_land = false;
   s_x = x;
   s_y = y;
   x_d_ = x_d;
   y_d_ = y_d;
   z_d_ = z_d;
end

== matlab function SIMULINK_ADP_Tracking_R2022b/CMD_UAV/CMD8/Subsystem/MATLAB Function ==
  settings: updateMethod=DISCRETE
  data: timestamp input; uavnum input; x_ output; y_ output; z_ output; switch_flag input; stas input; trj_flag input; form_flag input; avo_flag input
function [x_, y_, z_] = fcn(timestamp, uavnum,switch_flag,stas,trj_flag,form_flag,avo_flag)

[x_,y_,z_]=trjuav(timestamp,uavnum,switch_flag,stas,trj_flag,form_flag,avo_flag);

== matlab function SIMULINK_ADP_Tracking_R2022b/CMD_UAV/CMD10/MATLAB Function1 ==
  settings: updateMethod=DISCRETE
  data: x_d input; y_d input; z_d input; timestamp input; x input; y input; z input; battery_status input; sim_time_end input; x_d_ output; battery_threshold input; z_d_for_land input; y_d_ output; z_d_ output; UAV_NUM input
function [x_d_, y_d_, z_d_] = fcn(x_d, y_d, z_d, timestamp, x,y,z,battery_status, sim_time_end,battery_threshold, z_d_for_land, UAV_NUM)
persistent s_x s_y s_z ready_land
if isempty(s_x)
    s_x = x;
end
if isempty(s_y)
    s_y = y;
end
if isempty(s_z)
    s_z = z;
end
if isempty(ready_land)
    ready_land = false;
end
    
battery_low = false;
for i = 1:UAV_NUM
    if battery_status(i) < battery_threshold
        battery_low = true;
        break;
    end
end
if sim_time_end - timestamp < 1
    tello_stop = true;
else
    tello_stop = false;
end
if battery_low || tello_stop
    if ~ready_land
        ready_land = true;
    end
    z_d_ = z_d_for_land;
    x_d_ = s_x;
    y_d_ = s_y;
else
   ready_land = false;
   s_x = x;
   s_y = y;
   x_d_ = x_d;
   y_d_ = y_d;
   z_d_ = z_d;
end

== matlab function SIMULINK_ADP_Tracking_R2022b/CMD_UAV/CMD10/Subsystem/MATLAB Function ==
  settings: updateMethod=DISCRETE
  data: timestamp input; uavnum input; x_ output; y_ output; z_ output; switch_flag input; stas input; trj_flag input; form_flag input; avo_flag input
function [x_, y_, z_] = fcn(timestamp, uavnum,switch_flag,stas,trj_flag,form_flag,avo_flag)

[x_,y_,z_]=trjuav(timestamp,uavnum,switch_flag,stas,trj_flag,form_flag,avo_flag);

== matlab function SIMULINK_ADP_Tracking_R2022b/CMD_UAV/CMD9/MATLAB Function1 ==
  settings: updateMethod=DISCRETE
  data: x_d input; y_d input; z_d input; timestamp input; x input; y input; z input; battery_status input; sim_time_end input; x_d_ output; battery_threshold input; z_d_for_land input; y_d_ output; z_d_ output; UAV_NUM input
function [x_d_, y_d_, z_d_] = fcn(x_d, y_d, z_d, timestamp, x,y,z,battery_status, sim_time_end,battery_threshold, z_d_for_land, UAV_NUM)
persistent s_x s_y s_z ready_land
if isempty(s_x)
    s_x = x;
end
if isempty(s_y)
    s_y = y;
end
if isempty(s_z)
    s_z = z;
end
if isempty(ready_land)
    ready_land = false;
end
    
battery_low = false;
for i = 1:UAV_NUM
    if battery_status(i) < battery_threshold
        battery_low = true;
        break;
    end
end
if sim_time_end - timestamp < 1
    tello_stop = true;
else
    tello_stop = false;
end
if battery_low || tello_stop
    if ~ready_land
        ready_land = true;
    end
    z_d_ = z_d_for_land;
    x_d_ = s_x;
    y_d_ = s_y;
else
   ready_land = false;
   s_x = x;
   s_y = y;
   x_d_ = x_d;
   y_d_ = y_d;
   z_d_ = z_d;
end

== matlab function SIMULINK_ADP_Tracking_R2022b/CMD_UAV/CMD9/Subsystem/MATLAB Function ==
  settings: updateMethod=DISCRETE
  data: timestamp input; uavnum input; x_ output; y_ output; z_ output; switch_flag input; stas input; trj_flag input; form_flag input; avo_flag input
function [x_, y_, z_] = fcn(timestamp, uavnum,switch_flag,stas,trj_flag,form_flag,avo_flag)

[x_,y_,z_]=trjuav(timestamp,uavnum,switch_flag,stas,trj_flag,form_flag,avo_flag);

== matlab function SIMULINK_ADP_Tracking_R2022b/CMD_car1/CMD7/Subsystem/MATLAB Function ==
  settings: updateMethod=DISCRETE
  data: timestamp input; uavnum input; x_ output; y_ output; z_ output; switch_flag input; stas input; trj_flag input; form_flag input; avo_flag input
function [x_, y_, z_] = fcn(timestamp, uavnum,switch_flag,stas,trj_flag,form_flag,avo_flag)

[x_,y_,z_]=trjcar(timestamp,uavnum,switch_flag,stas,trj_flag,form_flag,avo_flag);

== matlab function SIMULINK_ADP_Tracking_R2022b/CMD_car1/CMD8/MATLAB Function1 ==
  settings: updateMethod=DISCRETE
  data: x_d input; y_d input; z_d input; timestamp input; x input; y input; z input; battery_status input; sim_time_end input; x_d_ output; battery_threshold input; z_d_for_land input; y_d_ output; z_d_ output; UAV_NUM input
function [x_d_, y_d_, z_d_] = fcn(x_d, y_d, z_d, timestamp, x,y,z,battery_status, sim_time_end,battery_threshold, z_d_for_land, UAV_NUM)
persistent s_x s_y s_z ready_land
if isempty(s_x)
    s_x = x;
end
if isempty(s_y)
    s_y = y;
end
if isempty(s_z)
    s_z = z;
end
if isempty(ready_land)
    ready_land = false;
end
    
battery_low = false;
for i = 1:UAV_NUM
    if battery_status(i) < battery_threshold
        battery_low = true;
        break;
    end
end
if sim_time_end - timestamp < 1
    tello_stop = true;
else
    tello_stop = false;
end
if battery_low || tello_stop
    if ~ready_land
        ready_land = true;
    end
    z_d_ = z_d_for_land;
    x_d_ = s_x;
    y_d_ = s_y;
else
   ready_land = false;
   s_x = x;
   s_y = y;
   x_d_ = x_d;
   y_d_ = y_d;
   z_d_ = z_d;
end

== matlab function SIMULINK_ADP_Tracking_R2022b/CMD_car1/CMD8/Subsystem/MATLAB Function ==
  settings: updateMethod=DISCRETE
  data: timestamp input; uavnum input; x_ output; y_ output; z_ output; switch_flag input; stas input; trj_flag input; form_flag input; avo_flag input
function [x_, y_, z_] = fcn(timestamp, uavnum,switch_flag,stas,trj_flag,form_flag,avo_flag)

[x_,y_,z_]=trjcar(timestamp,uavnum,switch_flag,stas,trj_flag,form_flag,avo_flag);
